simulink model "NL_PID_LC_MODEL"  (Simulink 7.6)
settings: Solver=ode45  StartTime=0.0  StopTime=20  RelTol=1e-3
settings Model: Creator=Administrator  LastModifiedBy=Administrator
settings DebuggingCC: SolverPrmCheckMsg=none

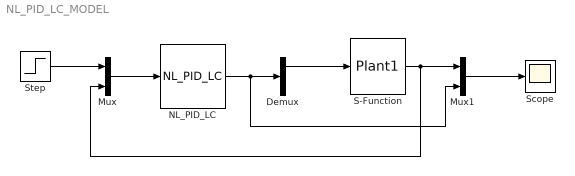
== system NL_PID_LC_MODEL ==
  Demux : Demux  Outputs=2
  Mux : Mux  Inputs=2
  Mux1 : Mux  Inputs=2
  NL_PID_LC : S-Function  FunctionName=NL_PID_LC  Parameters=r0,h0,r1,h1,h,Bet  EnableBusSupport=off  mask{r0=0.5, h0=0.01, r1=30, h1=0.01, h=0.01, Bet=[50,80,30]}
      mask prompts: r0 "r0="; h0 "h0="; r1 "r1="; h1 "h1="; h "h="; Bet "Bet=[ ; ; ]"
  S-Function : S-Function  FunctionName=Plant1  EnableBusSupport=off
  Scope : Scope
      settings: YMin=0  YMax=2
  Step : Step  Time=0  SampleTime=0
  wires:
  Mux/1 -> NL_PID_LC/1
  Step/1 -> Mux/1
  S-Function/1 -> Mux/2, Mux1/1
  Mux1/1 -> Scope/1
  NL_PID_LC/1 -> Demux/1, Mux1/2
  Demux/1 -> S-Function/1
